simulink model "DynamicEDFAs"  (Simulink 4.00)
settings: Solver=FixedStepDiscrete  StartTime=0.0  StopTime=0.0005  FixedStep=0.0000005  RelTol=1e-3
settings Model: LastModifiedBy=Andres  MaxDataPoints=100000  RTWOptions="-aEnforceIntegerDowncast=1 -aExtMode=0 -aFoldNonRolledExpr=1 -aForceParamTrailComments=0 -aGenerateComments=1 -aIgnoreCustomStorageClasses=0 -aIncHierarchyInIds=0 -aInlineInvariantSignals=0 -aLocalBlockOutputs=1 -aLogVarNameModifier=\"rt_\" -aRTWVerbose=1 -aRollThreshold=5 -aShowEliminatedStatements=1"

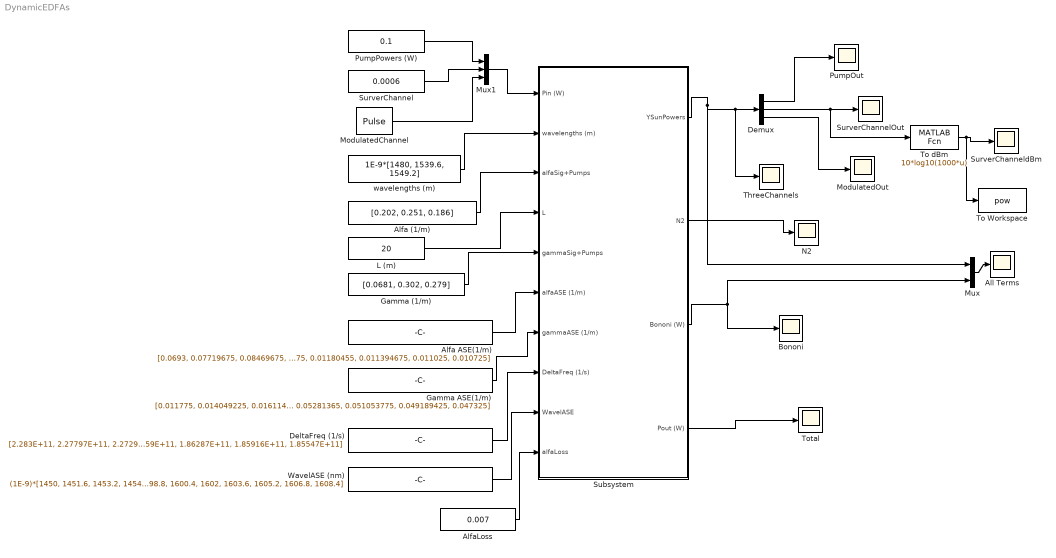
== system DynamicEDFAs ==
  Alfa (1/m) : Constant  Value=[0.202, 0.251, 0.186]
  Alfa ASE(1/m) : Constant  Value=[0.0693, 0.07719675, 0.08469675, 0.0902955, 0.10103775, 0.1092345, 0.118182, 0.12543975, 0.13178775, 0.13880475, 0.14496975, 0.15233325, 0.159432, 0.16653, 0.17287875, 0.17995425, 0.1855755, 0.19192425, 0.196773, 0.201621, 0.20721975, 0.2113185, 0.2145, 0.21726525, 0.219864, 0.22275, 0.225, 0.22575, 0.22725, 0.228, 0.228, 0.22875, 0.2295, 0.231, 0.2323485, 0.23514375, 0.23979525, 0.246288, 0.25099275, 0.25809075, 0.2653185, 0.276864, 0.28990875, 0.30818925, 0.33350025, 0.36259125, 0.39262125, 0.42140175, 0.4332045, 0.44025, 0.43540125, 0.41272725, 0.36203025, 0.31630275, 0.2796135, 0.26124975, 0.251235, 0.24038625, 0.23107575, 0.219129, 0.2079315, 0.19699275, 0.186288, 0.17659125, 0.16764375, 0.160947, 0.15200025, 0.14305275, 0.134106, 0.12365925, 0.112818, 0.102015, 0.09156825, 0.0811215, 0.071499225, 0.0625818, 0.05482425, 0.048875025, 0.04371135, 0.0394977, 0.03598485, 0.032440875, 0.029602275, 0.027505275, 0.025715925, 0.0238515, 0.022134075, 0.020529525, 0.019149975, 0.017545425, 0.0164523, 0.01548255, 0.014587875, 0.0137682, 0.01287345, 0.012353775, 0.01180455, 0.011394675, 0.011025, 0.010725]
  AlfaLoss : Constant  Value=0.007
  All Terms : Scope
      settings: TimeRange=auto  YMin=-5  YMax=5  SaveToWorkspace=off  SaveName=ScopeData6  LimitDataPoints=on  MaxDataPoints=5000
  Bononi : Scope
      settings: TimeRange=auto  YMin=-5  YMax=5  SaveToWorkspace=off  SaveName=ScopeData4  LimitDataPoints=on  MaxDataPoints=5000
  DeltaFreq (1/s) : Constant  Value=[2.283E+11, 2.27797E+11, 2.27295E+11, 2.26796E+11, 2.26298E+11, 2.25801E+11, 2.25306E+11, 2.24813E+11, 2.24322E+11, 2.23832E+11, 2.23343E+11, 2.22857E+11, 2.22372E+11, 2.21888E+11, 2.21406E+11, 2.20926E+11, 2.20447E+11, 2.1997E+11, 2.19494E+11, 2.1902E+11, 2.18547E+11, 2.18076E+11, 2.17606E+11, 2.17138E+11, 2.16672E+11, 2.16206E+11, 2.15743E+11, 2.15281E+11, 2.1482E+11, 2.14361E+11, 2.13903E+11, 2.13447E+11, 2.12992E+11, 2.12539E+11, 2.12087E+11, 2.11637E+11, 2.11188E+11, 2.1074E+11, 2.10294E+11, 2.09849E+11, 2.09406E+11, 2.08964E+11, 2.08524E+11, 2.08085E+11, 2.07647E+11, 2.07211E+11, 2.06776E+11, 2.06342E+11, 2.0591E+11, 2.05479E+11, 2.05049E+11, 2.04621E+11, 2.04194E+11, 2.03769E+11, 2.03345E+11, 2.02922E+11, 2.025E+11, 2.0208E+11, 2.01661E+11, 2.01243E+11, 2.00827E+11, 2.00412E+11, 1.99998E+11, 1.99586E+11, 1.99175E+11, 1.98765E+11, 1.98356E+11, 1.97949E+11, 1.97542E+11, 1.97138E+11, 1.96734E+11, 1.96331E+11, 1.9593E+11, 1.9553E+11, 1.95132E+11, 1.94734E+11, 1.94338E+11, 1.93943E+11, 1.93549E+11, 1.93156E+11, 1.92765E+11, 1.92374E+11, 1.91985E+11, 1.91597E+11, 1.9121E+11, 1.90825E+11, 1.9044E+11, 1.90057E+11, 1.89675E+11, 1.89294E+11, 1.88914E+11, 1.88536E+11, 1.88158E+11, 1.87782E+11, 1.87406E+11, 1.87032E+11, 1.86659E+11, 1.86287E+11, 1.85916E+11, 1.85547E+11]
  Demux : Demux  Outputs=3  BusSelectionMode=off
  Gamma (1/m) : Constant  Value=[0.0681, 0.302, 0.279]
  Gamma ASE(1/m) : Constant  Value=[0.011775, 0.014049225, 0.016114425, 0.0172341, 0.020796975, 0.022974225, 0.02325, 0.0261576, 0.029272725, 0.033096825, 0.0357924, 0.0382917, 0.040834125, 0.0445773, 0.049015875, 0.053379525, 0.057335625, 0.061356825, 0.064765875, 0.06814695, 0.072263625, 0.0778185, 0.0826665, 0.08676525, 0.09075, 0.094962, 0.09975, 0.10315875, 0.1080075, 0.11210625, 0.11620425, 0.121803, 0.12590175, 0.13074975, 0.1363485, 0.14364375, 0.15204525, 0.160644, 0.16973475, 0.1794315, 0.1910685, 0.207114, 0.22429575, 0.24668925, 0.27683325, 0.31220475, 0.349962, 0.38890875, 0.41363625, 0.43447725, 0.4395, 0.42743175, 0.39353025, 0.355212, 0.321477, 0.30549975, 0.3015, 0.30038625, 0.29782575, 0.2951895, 0.29034075, 0.28523475, 0.278682, 0.27204525, 0.26794725, 0.2645985, 0.26049975, 0.25565175, 0.247803, 0.23615925, 0.223068, 0.2092725, 0.193977, 0.1771815, 0.161136, 0.14584125, 0.13204575, 0.121083, 0.11213625, 0.1039395, 0.09799275, 0.091773, 0.08625, 0.0828255, 0.0802275, 0.07687875, 0.07374315, 0.071090925, 0.068600025, 0.065765925, 0.063054525, 0.061115175, 0.05938185, 0.0581364, 0.056121975, 0.054075, 0.05281365, 0.051053775, 0.049189425, 0.047325]
  L (m) : Constant  Value=20
  ModulatedChannel : DiscretePulseGenerator  PulseType=Time-based  Amplitude=0.0018  Period=0.0005  PulseWidth=50  PhaseDelay=0  SampleTime=1
  ModulatedOut : Scope
      settings: TimeRange=0.05  YMin=0  YMax=0.1  SaveToWorkspace=off  SaveName=ScopeData  LimitDataPoints=on  MaxDataPoints=5000
  Mux : Mux  Inputs=2
  Mux1 : Mux  Inputs=3
  N2 : Scope
      settings: TimeRange=auto  YMin=-5  YMax=5  SaveToWorkspace=off  LimitDataPoints=on  MaxDataPoints=5000
  PumpOut : Scope
      settings: TimeRange=0.05  YMin=0  YMax=0.08  SaveToWorkspace=off  SaveName=ScopeData3  LimitDataPoints=on  MaxDataPoints=5000
  PumpPowers (W) : Constant  Value=0.1
  Subsystem : Subsystem
      settings: RTWFcnNameOpts=Auto  RTWFileNameOpts=Auto
  SurverChannel : Constant  Value=0.0006
  SurverChannelOut : Scope
      settings: TimeRange=0.05  YMin=0  YMax=0.08  SaveToWorkspace=off  SaveName=ScopeData9  LimitDataPoints=on  MaxDataPoints=5000
  SurverChanneldBm : Scope
      settings: TimeRange=0.05  YMin=0  YMax=0.08  SaveToWorkspace=off  SaveName=ScopeData12  LimitDataPoints=on  MaxDataPoints=5000
  ThreeChannels : Scope
      settings: TimeRange=0.05  YMin=0  YMax=0.1  SaveToWorkspace=off  SaveName=ScopeData10  LimitDataPoints=on  MaxDataPoints=5000
  To Workspace : ToWorkspace  VariableName=pow  SampleTime=-1  SaveFormat=Array
  To dBm : MATLABFcn  MATLABFcn=10*log10(1000*u)  OutputDimensions=1  OutputSignalType=auto  Output1D=on
  Total : Scope
      settings: TimeRange=auto  YMin=-5  YMax=5  SaveToWorkspace=off  SaveName=ScopeData5  LimitDataPoints=on  MaxDataPoints=5000
  WavelASE (nm) : Constant  Value=(1E-9)*[1450, 1451.6, 1453.2, 1454.8, 1456.4, 1458, 1459.6, 1461.2, 1462.8, 1464.4, 1466, 1467.6, 1469.2, 1470.8, 1472.4, 1474, 1475.6, 1477.2, 1478.8, 1480.4, 1482, 1483.6, 1485.2, 1486.8, 1488.4, 1490, 1491.6, 1493.2, 1494.8, 1496.4, 1498, 1499.6, 1501.2, 1502.8, 1504.4, 1506, 1507.6, 1509.2, 1510.8, 1512.4, 1514, 1515.6, 1517.2, 1518.8, 1520.4, 1522, 1523.6, 1525.2, 1526.8, 1528.4, 1530, 1531.6, 1533.2, 1534.8, 1536.4, 1538, 1539.6, 1541.2, 1542.8, 1544.4, 1546, 1547.6, 1549.2, 1550.8, 1552.4, 1554, 1555.6, 1557.2, 1558.8, 1560.4, 1562, 1563.6, 1565.2, 1566.8, 1568.4, 1570, 1571.6, 1573.2, 1574.8, 1576.4, 1578, 1579.6, 1581.2, 1582.8, 1584.4, 1586, 1587.6, 1589.2, 1590.8, 1592.4, 1594, 1595.6, 1597.2, 1598.8, 1600.4, 1602, 1603.6, 1605.2, 1606.8, 1608.4]
  wavelengths (m) : Constant  Value=1E-9*[1480, 1539.6, 1549.2]
  wires:
  Subsystem/1(YSunPowers) -> Mux/1, Demux/1, ThreeChannels/1
  Subsystem/2(N2) -> N2/1
  Alfa (1/m)/1 -> Subsystem/3("alfaSig+Pumps ")
  L (m)/1 -> Subsystem/4(L)
  Gamma (1/m)/1 -> Subsystem/5(gammaSig+Pumps)
  wavelengths (m)/1 -> Subsystem/2(wavelengths (m))
  Gamma ASE(1/m)/1 -> Subsystem/7(gammaASE (1/m))
  DeltaFreq (1/s)/1 -> Subsystem/8(DeltaFreq (1/s))
  Alfa ASE(1/m)/1 -> Subsystem/6(alfaASE (1/m))
  WavelASE (nm)/1 -> Subsystem/9(WavelASE)
  Subsystem/3(Bononi (W)) -> Bononi/1, Mux/2
  Subsystem/4(Pout (W)) -> Total/1
  Mux/1 -> All Terms/1
  AlfaLoss/1 -> Subsystem/10(alfaLoss)
  PumpPowers (W)/1 -> Mux1/1
  SurverChannel/1 -> Mux1/2
  ModulatedChannel/1 -> Mux1/3
  Mux1/1 -> Subsystem/1(Pin (W))
  Demux/1 -> PumpOut/1
  Demux/2 -> SurverChannelOut/1, To dBm/1
  Demux/3 -> ModulatedOut/1
  To dBm/1 -> SurverChanneldBm/1, To Workspace/1

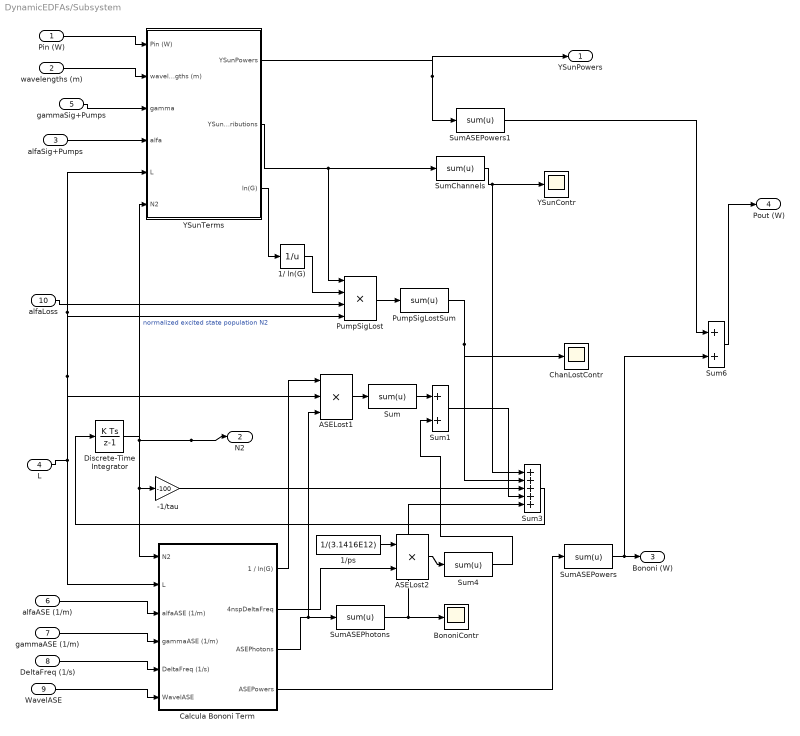
== system DynamicEDFAs/Subsystem ==
  Pin (W) : Inport  Port=1  LatchInput=off
  wavelengths (m) : Inport  Port=2  LatchInput=off
  "alfaSig+Pumps " : Inport  Port=3  LatchInput=off
  L : Inport  Port=4  LatchInput=off
  gammaSig+Pumps : Inport  Port=5  LatchInput=off
  alfaASE (1/m) : Inport  Port=6  LatchInput=off
  gammaASE (1/m) : Inport  Port=7  LatchInput=off
  DeltaFreq (1/s) : Inport  Port=8  LatchInput=off
  WavelASE : Inport  Port=9  LatchInput=off
  alfaLoss : Inport  Port=10  LatchInput=off
  -1/tau : Gain  Gain=-100  Multiplication=Element-wise(K.*u)  SaturateOnIntegerOverflow=on
  1/ ln(G) : Math  Operator=reciprocal  OutputSignalType=auto
  1/ps : Constant  Value=1/(3.1416E12)
  ASELost1 : Product  Inputs=3  Multiplication=Element-wise(.*)  SaturateOnIntegerOverflow=on
  ASELost2 : Product  Inputs=2  Multiplication=Element-wise(.*)  SaturateOnIntegerOverflow=on
  BononiContr : Scope
      settings: TimeRange=auto  YMin=-5  YMax=5  SaveToWorkspace=off  SaveName=ScopeData8  LimitDataPoints=on  MaxDataPoints=5000
  Calcula Bononi Term : Subsystem
      settings: RTWFcnNameOpts=Auto  RTWFileNameOpts=Auto
      mask Type: Bononi Term
  ChanLostContr : Scope
      settings: TimeRange=auto  YMin=-5  YMax=5  SaveToWorkspace=off  SaveName=ScopeData11  LimitDataPoints=on  MaxDataPoints=5000
  Discrete-Time Integrator : DiscreteIntegrator  IntegratorMethod=ForwardEuler  ExternalReset=none  InitialConditionSource=internal  InitialCondition=0.7  LimitOutput=off  UpperSaturationLimit=inf  LowerSaturationLimit=-inf  ShowSaturationPort=off  ShowStatePort=off  SampleTime=-1
      settings: RTWStateStorageClass=Auto
  PumpSigLost : Product  Inputs=4  Multiplication=Element-wise(.*)  SaturateOnIntegerOverflow=on
  PumpSigLostSum : MATLABFcn  MATLABFcn=sum(u)  OutputDimensions=1  OutputSignalType=auto  Output1D=on
  Sum : MATLABFcn  MATLABFcn=sum(u)  OutputDimensions=1  OutputSignalType=auto  Output1D=on
  Sum1 : Sum  Inputs=++  SaturateOnIntegerOverflow=on
  Sum3 : Sum  Inputs=+++++  SaturateOnIntegerOverflow=on
  Sum4 : MATLABFcn  MATLABFcn=sum(u)  OutputDimensions=1  OutputSignalType=auto  Output1D=on
  Sum6 : Sum  Inputs=++  SaturateOnIntegerOverflow=on
  SumASEPhotons : MATLABFcn  MATLABFcn=sum(u)  OutputDimensions=1  OutputSignalType=auto  Output1D=on
  SumASEPowers : MATLABFcn  MATLABFcn=sum(u)  OutputDimensions=1  OutputSignalType=auto  Output1D=on
  SumASEPowers1 : MATLABFcn  MATLABFcn=sum(u)  OutputDimensions=1  OutputSignalType=auto  Output1D=on
  SumChannels : MATLABFcn  MATLABFcn=sum(u)  OutputDimensions=1  OutputSignalType=auto  Output1D=on
  YSunContr : Scope
      settings: TimeRange=auto  YMin=-5  YMax=5  SaveToWorkspace=off  SaveName=ScopeData7  LimitDataPoints=on  MaxDataPoints=5000
  YSunTerms : Subsystem
      settings: RTWFcnNameOpts=Auto  RTWFileNameOpts=Auto
  YSunPowers : Outport  Port=1
  N2 : Outport  Port=2
  Bononi (W) : Outport  Port=3
  Pout (W) : Outport  Port=4
  wires:
  Discrete-Time Integrator/1 -> Calcula Bononi Term/1(N2), -1/tau/1, YSunTerms/6(N2), N2/1  "normalized excited state population N2"
  Sum3/1 -> Discrete-Time Integrator/1
  Sum6/1 -> Pout (W)/1
  SumASEPowers/1 -> Sum6/2, Bononi (W)/1
  SumASEPowers1/1 -> Sum6/1
  Calcula Bononi Term/4(ASEPowers) -> SumASEPowers/1
  alfaASE (1/m)/1 -> Calcula Bononi Term/3(alfaASE (1/m))
  gammaASE (1/m)/1 -> Calcula Bononi Term/4(gammaASE (1/m))
  DeltaFreq (1/s)/1 -> Calcula Bononi Term/5(DeltaFreq (1/s))
  WavelASE/1 -> Calcula Bononi Term/6(WavelASE)
  Pin (W)/1 -> YSunTerms/1(Pin (W))
  wavelengths (m)/1 -> YSunTerms/2(wavelengths (m))
  "alfaSig+Pumps "/1 -> YSunTerms/4("alfa ")
  L/1 -> Calcula Bononi Term/2(L), YSunTerms/5(L), PumpSigLost/4, ASELost1/2
  gammaSig+Pumps/1 -> YSunTerms/3(gamma)
  YSunTerms/1(YSunPowers) -> SumASEPowers1/1, YSunPowers/1
  SumChannels/1 -> Sum3/1, YSunContr/1
  YSunTerms/2(YSunContributions) -> SumChannels/1, PumpSigLost/1
  YSunTerms/3(ln(G)) -> 1/ ln(G)/1
  1/ ln(G)/1 -> PumpSigLost/2
  -1/tau/1 -> Sum3/3
  alfaLoss/1 -> PumpSigLost/3
  PumpSigLost/1 -> PumpSigLostSum/1
  PumpSigLostSum/1 -> Sum3/2, ChanLostContr/1
  1/ps/1 -> ASELost2/1
  ASELost1/1 -> Sum/1
  Sum/1 -> Sum1/1
  ASELost2/1 -> Sum4/1
  Sum4/1 -> Sum1/2
  SumASEPhotons/1 -> BononiContr/1, Sum3/5
  Calcula Bononi Term/1(1 / ln(G)) -> ASELost1/1
  Calcula Bononi Term/2(4nspDeltaFreq) -> ASELost2/2
  Calcula Bononi Term/3(ASEPhotons) -> SumASEPhotons/1, ASELost1/3
  Sum1/1 -> Sum3/4

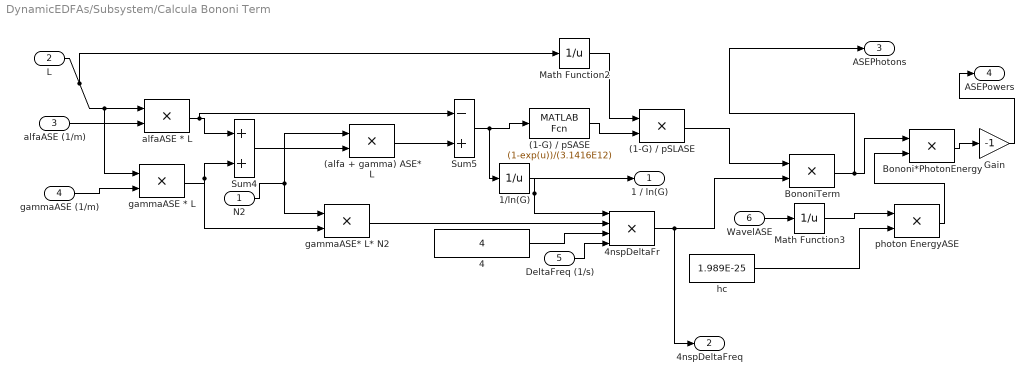
== system DynamicEDFAs/Subsystem/Calcula Bononi Term ==
  N2 : Inport  Port=1  LatchInput=off
  L : Inport  Port=2  LatchInput=off
  alfaASE (1/m) : Inport  Port=3  LatchInput=off
  gammaASE (1/m) : Inport  Port=4  LatchInput=off
  DeltaFreq (1/s) : Inport  Port=5  LatchInput=off
  WavelASE : Inport  Port=6  LatchInput=off
  (1-G) / pSASE : MATLABFcn  MATLABFcn=(1-exp(u))/(3.1416E12)  OutputDimensions=100  OutputSignalType=auto  Output1D=off
  (1-G) / pSLASE : Product  Inputs=2  Multiplication=Element-wise(.*)  SaturateOnIntegerOverflow=on
  (alfa + gamma) ASE* L : Product  Inputs=2  Multiplication=Element-wise(.*)  SaturateOnIntegerOverflow=on
  1/ln(G) : Math  Operator=reciprocal  OutputSignalType=auto
  4 : Constant  Value=4
  4nspDeltaFr : Product  Inputs=4  Multiplication=Element-wise(.*)  SaturateOnIntegerOverflow=on
  Bononi*PhotonEnergy : Product  Inputs=2  Multiplication=Element-wise(.*)  SaturateOnIntegerOverflow=on
  BononiTerm : Product  Inputs=2  Multiplication=Element-wise(.*)  SaturateOnIntegerOverflow=on
  Gain : Gain  Gain=-1  Multiplication=Element-wise(K.*u)  SaturateOnIntegerOverflow=on
  Math Function2 : Math  Operator=reciprocal  OutputSignalType=auto
  Math Function3 : Math  Operator=reciprocal  OutputSignalType=auto
  Sum4 : Sum  Inputs=++  SaturateOnIntegerOverflow=on
  Sum5 : Sum  Inputs=-+  SaturateOnIntegerOverflow=on
  alfaASE * L : Product  Inputs=2  Multiplication=Element-wise(.*)  SaturateOnIntegerOverflow=on
  gammaASE * L : Product  Inputs=2  Multiplication=Element-wise(.*)  SaturateOnIntegerOverflow=on
  "gammaASE* L* N2 " : Product  Inputs=2  Multiplication=Element-wise(.*)  SaturateOnIntegerOverflow=on
  hc : Constant  Value=1.989E-25
  photon EnergyASE : Product  Inputs=2  Multiplication=Element-wise(.*)  SaturateOnIntegerOverflow=on
  1 / ln(G) : Outport  Port=1
  4nspDeltaFreq : Outport  Port=2
  ASEPhotons : Outport  Port=3
  ASEPowers : Outport  Port=4
  wires:
  alfaASE (1/m)/1 -> alfaASE * L/2
  gammaASE (1/m)/1 -> gammaASE * L/2
  alfaASE * L/1 -> Sum4/1, Sum5/1
  gammaASE * L/1 -> Sum4/2, "gammaASE* L* N2 "/2
  Sum4/1 -> (alfa + gamma) ASE* L/2
  (alfa + gamma) ASE* L/1 -> Sum5/2
  Sum5/1 -> (1-G) / pSASE/1, 1/ln(G)/1
  "gammaASE* L* N2 "/1 -> 4nspDeltaFr/2
  1/ln(G)/1 -> 4nspDeltaFr/1, 1 / ln(G)/1
  DeltaFreq (1/s)/1 -> 4nspDeltaFr/4
  4/1 -> 4nspDeltaFr/3
  4nspDeltaFr/1 -> BononiTerm/2, 4nspDeltaFreq/1
  BononiTerm/1 -> Bononi*PhotonEnergy/1, ASEPhotons/1
  photon EnergyASE/1 -> Bononi*PhotonEnergy/2
  WavelASE/1 -> Math Function3/1
  hc/1 -> photon EnergyASE/2
  Math Function3/1 -> photon EnergyASE/1
  (1-G) / pSASE/1 -> (1-G) / pSLASE/2
  (1-G) / pSLASE/1 -> BononiTerm/1
  L/1 -> alfaASE * L/1, gammaASE * L/1, Math Function2/1
  N2/1 -> (alfa + gamma) ASE* L/1, "gammaASE* L* N2 "/1
  Math Function2/1 -> (1-G) / pSLASE/1
  Bononi*PhotonEnergy/1 -> Gain/1
  Gain/1 -> ASEPowers/1

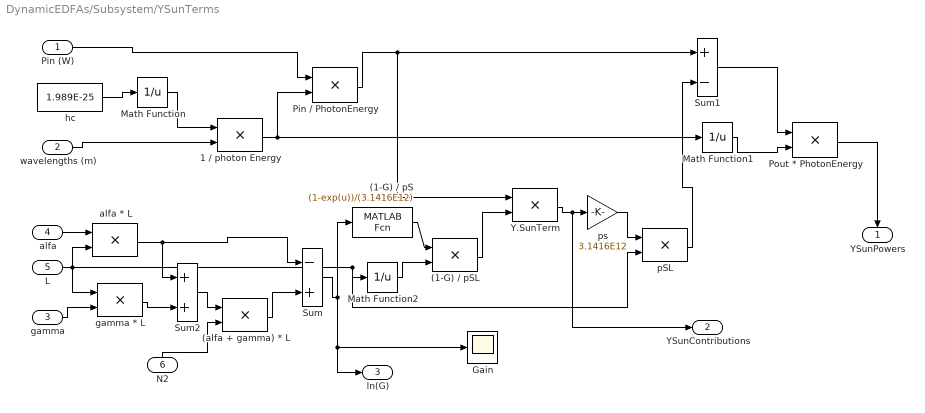
== system DynamicEDFAs/Subsystem/YSunTerms ==
  Pin (W) : Inport  Port=1  LatchInput=off
  wavelengths (m) : Inport  Port=2  LatchInput=off
  gamma : Inport  Port=3  LatchInput=off
  "alfa " : Inport  Port=4  LatchInput=off
  L : Inport  Port=5  LatchInput=off
  N2 : Inport  Orientation=up  Port=6  LatchInput=off
  (1-G) / pS : MATLABFcn  MATLABFcn=(1-exp(u))/(3.1416E12)  OutputDimensions=3  OutputSignalType=auto  Output1D=off
  (1-G) / pSL : Product  Inputs=2  Multiplication=Element-wise(.*)  SaturateOnIntegerOverflow=on
  (alfa + gamma) * L : Product  Inputs=2  Multiplication=Element-wise(.*)  SaturateOnIntegerOverflow=on
  1 / photon Energy : Product  Inputs=2  Multiplication=Element-wise(.*)  SaturateOnIntegerOverflow=on
  Gain : Scope
      settings: TimeRange=auto  YMin=-5  YMax=5  SaveToWorkspace=off  SaveName=ScopeData2  LimitDataPoints=on  MaxDataPoints=5000
  Math Function : Math  Operator=reciprocal  OutputSignalType=auto
  Math Function1 : Math  Operator=reciprocal  OutputSignalType=auto
  Math Function2 : Math  Operator=reciprocal  OutputSignalType=auto
  Pin / PhotonEnergy : Product  Inputs=2  Multiplication=Element-wise(.*)  SaturateOnIntegerOverflow=on
  Pout * PhotonEnergy : Product  Inputs=2  Multiplication=Element-wise(.*)  SaturateOnIntegerOverflow=on
  Sum : Sum  Inputs=-+  SaturateOnIntegerOverflow=on
  Sum1 : Sum  Inputs=+-  SaturateOnIntegerOverflow=on
  Sum2 : Sum  Inputs=++  SaturateOnIntegerOverflow=on
  Y.SunTerm : Product  Inputs=2  Multiplication=Element-wise(.*)  SaturateOnIntegerOverflow=on
  alfa * L : Product  Inputs=2  Multiplication=Element-wise(.*)  SaturateOnIntegerOverflow=on
  gamma * L : Product  Inputs=2  Multiplication=Element-wise(.*)  SaturateOnIntegerOverflow=on
  "hc " : Constant  Value=1.989E-25
  pSL : Product  Inputs=2  Multiplication=Element-wise(.*)  SaturateOnIntegerOverflow=on
  ps : Gain  Gain=3.1416E12  Multiplication=Element-wise(K.*u)  SaturateOnIntegerOverflow=on
  YSunPowers : Outport  Orientation=down  Port=1
  YSunContributions : Outport  Port=2
  ln(G) : Outport  Port=3
  wires:
  Y.SunTerm/1 -> ps/1, YSunContributions/1
  alfa * L/1 -> Sum/1, Sum2/1
  (alfa + gamma) * L/1 -> Sum/2
  Sum/1 -> (1-G) / pS/1, Gain/1, ln(G)/1
  Pin (W)/1 -> Pin / PhotonEnergy/1
  Sum1/1 -> Pout * PhotonEnergy/1
  "alfa "/1 -> alfa * L/1
  L/1 -> alfa * L/2, gamma * L/1, Math Function2/1, pSL/2
  gamma/1 -> gamma * L/2
  gamma * L/1 -> Sum2/2
  Sum2/1 -> (alfa + gamma) * L/1
  Pin / PhotonEnergy/1 -> Sum1/1, Y.SunTerm/1
  "hc "/1 -> Math Function/1
  wavelengths (m)/1 -> 1 / photon Energy/2
  Math Function/1 -> 1 / photon Energy/1
  1 / photon Energy/1 -> Pin / PhotonEnergy/2, Math Function1/1
  Math Function1/1 -> Pout * PhotonEnergy/2
  (1-G) / pS/1 -> (1-G) / pSL/1
  Math Function2/1 -> (1-G) / pSL/2
  (1-G) / pSL/1 -> Y.SunTerm/2
  N2/1 -> (alfa + gamma) * L/2
  Pout * PhotonEnergy/1 -> YSunPowers/1
  ps/1 -> pSL/1
  pSL/1 -> Sum1/2
